simulink model "nav22"  (R2020a)
settings: Solver=VariableStepAuto  StartTime=0.0  StopTime=inf  RelTol=1e-3
values from neighbouring files (symbols this model uses):
  chargingStn = [3, 2]    [startup.m]
  L2RTransform = [cos(L2Rtheta), -sin(L2Rtheta), L2Rx ... (first row only)    [startup.m]
  LIVE_MODE = 1    [startup.m]
  loadingStn = [4, 3]    [startup.m]
  logicalMap = simMapPad < 100    [startup.m]
  unloadingStn = [15, 15]    [startup.m]
  W2LOTransform = W2ORTransform/(L2RTransform)    [startup.m]
  wheelBase = 0.4464    [startup.m]
  wheelRadius = 0.1715/2    (= 0.08575)    [startup.m]
undefined symbols (not defined in the file or in its folder): Angular, Linear
libraries: robotlib x6, robotalgslib x1
settings Model: EnablePacing=on  Creator=john  LastModifiedBy=john

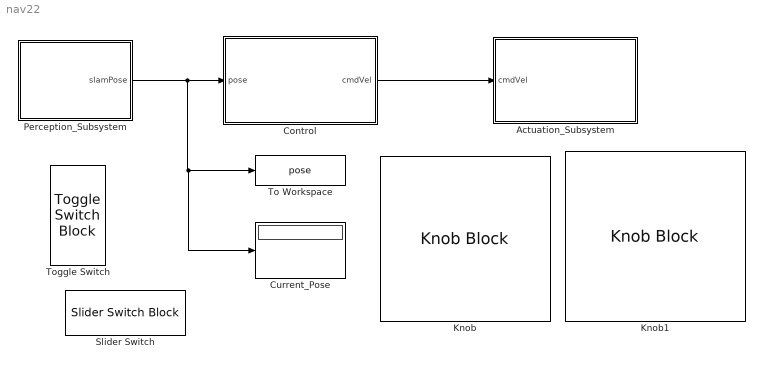
== system nav22 ==
  Actuation_Subsystem : Subsystem
  Control : Subsystem
  Current_Pose : Display
  Knob : KnobBlock  ScaleMin=-5  ScaleMax=5
  Knob1 : KnobBlock  ScaleMin=-1  ScaleMax=1
  Perception_Subsystem : Subsystem
  Slider Switch : SliderSwitchBlock
      settings: Values={{'Off', 'On'}, [0 1]}
  To Workspace : ToWorkspace  VariableName=pose  SaveFormat=Timeseries  SampleTime=-1
  Toggle Switch : ToggleSwitchBlock
      settings: Values={{'Off', 'On'}, [1 0]}
  wires:
  Perception_Subsystem/1(slamPose) -> Current_Pose/1, To Workspace/1, Control/1(pose)
  Control/1(cmdVel) -> Actuation_Subsystem/1(cmdVel)

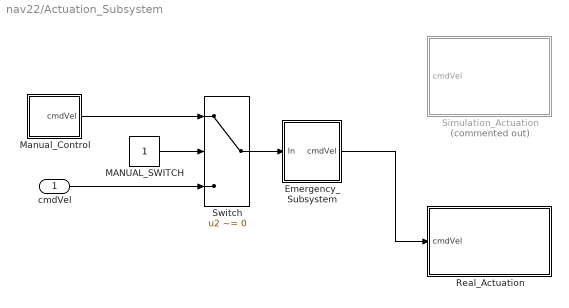
== system nav22/Actuation_Subsystem ==
  cmdVel : Inport
  Emergency_Subsystem : Subsystem
  MANUAL_SWITCH : Constant
  Manual_Control : Subsystem
  Real_Actuation : Subsystem
  Simulation_Actuation : Subsystem  Commented=on
  Switch : Switch  Criteria=u2 ~= 0
  wires:
  cmdVel/1 -> Switch/3
  Manual_Control/1(cmdVel) -> Switch/1
  Switch/1 -> Emergency_Subsystem/1(In)
  Emergency_Subsystem/1(cmdVel) -> Real_Actuation/1(cmdVel)
  MANUAL_SWITCH/1 -> Switch/2

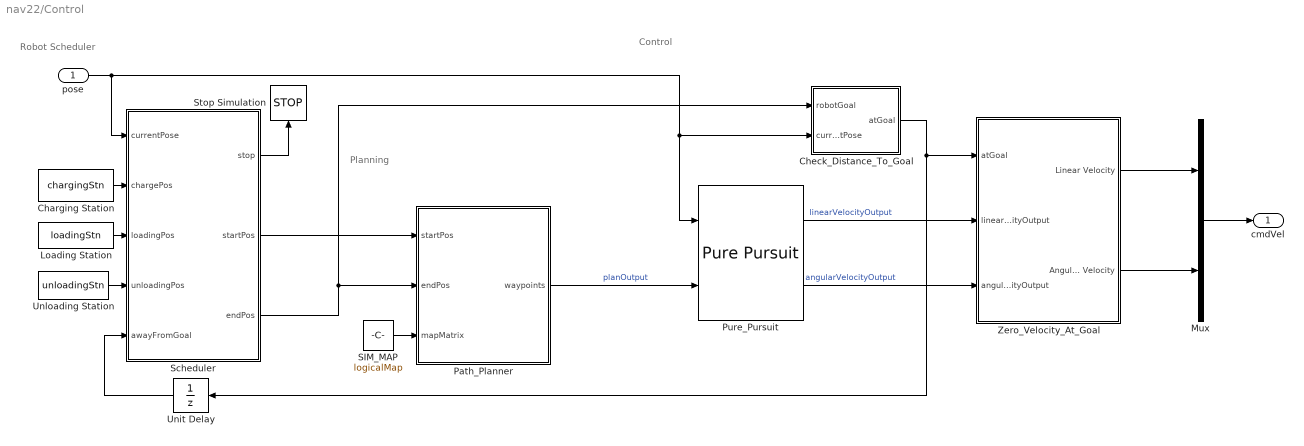
== system nav22/Control ==
  note: Control
  note: Robot Scheduler
  note: Planning
  pose : Inport
  "Charging Station " : Constant  Value=chargingStn  SampleTime=1
  Check_Distance_To_Goal : Subsystem
  Loading Station : Constant  Value=loadingStn
  Mux : Mux  Inputs=2
  Path_Planner : MATLAB Function  TreatAsAtomicUnit=on
  Pure_Pursuit : robotalgslib/Pure Pursuit  DesiredLinearVelocity=1  MaxAngularVelocity=0.5  LookaheadDistance=1  TargetDirPort=off  SimulateUsing=Code generation
  SIM_MAP : Constant  Value=logicalMap  SampleTime=1
  Scheduler : Stateflow chart  TreatAsAtomicUnit=on
  Stop Simulation : Stop
  Unit Delay : UnitDelay  SampleTime=-1  HasFrameUpgradeWarning=on
  Unloading Station : Constant  Value=unloadingStn  SampleTime=1
  Zero_Velocity_At_Goal : Subsystem
  cmdVel : Outport
  wires:
  Check_Distance_To_Goal/1(atGoal) -> Unit Delay/1, Zero_Velocity_At_Goal/1(atGoal)
  "Charging Station "/1 -> Scheduler/2(chargePos)
  Scheduler/2(startPos) -> Path_Planner/1(startPos)
  Unit Delay/1 -> Scheduler/5(awayFromGoal)
  Scheduler/3(endPos) -> Path_Planner/2(endPos), Check_Distance_To_Goal/1(robotGoal)
  Loading Station/1 -> Scheduler/3(loadingPos)
  Pure_Pursuit/2 -> Zero_Velocity_At_Goal/3(angularVelocityOutput)  "angularVelocityOutput"
  pose/1 -> Check_Distance_To_Goal/2(currentPose), Pure_Pursuit/1, Scheduler/1(currentPose)
  Unloading Station/1 -> Scheduler/4(unloadingPos)
  Scheduler/1(stop) -> Stop Simulation/1
  Path_Planner/1(waypoints) -> Pure_Pursuit/2  "planOutput"
  Pure_Pursuit/1 -> Zero_Velocity_At_Goal/2(linearVelocityOutput)  "linearVelocityOutput"
  Zero_Velocity_At_Goal/2(Angular Velocity) -> Mux/2
  Zero_Velocity_At_Goal/1(Linear Velocity) -> Mux/1
  Mux/1 -> cmdVel/1
  SIM_MAP/1 -> Path_Planner/3(mapMatrix)

== system nav22/Perception_Subsystem ==
  SLAM_Subsystem : Subsystem
  slamPose : Outport
  wires:
  SLAM_Subsystem/1(slamPose) -> slamPose/1

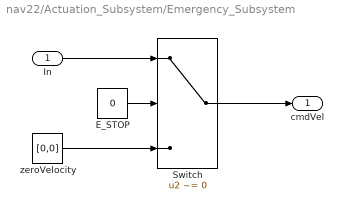
== system nav22/Actuation_Subsystem/Emergency_Subsystem ==
  In : Inport
  E_STOP : Constant  Value=0
  Switch : Switch  Criteria=u2 ~= 0  Threshold=1
  zeroVelocity : Constant  Value=[0,0]
  cmdVel : Outport
  wires:
  Switch/1 -> cmdVel/1
  E_STOP/1 -> Switch/2
  In/1 -> Switch/1
  zeroVelocity/1 -> Switch/3

== system nav22/Actuation_Subsystem/Manual_Control ==
  Mux : Mux  Inputs=2
  angularVel : Constant  Value=-0.007065188519232657
  linearVel : Constant  Value=2.054641124404234
  cmdVel : Outport
  wires:
  linearVel/1 -> Mux/1
  angularVel/1 -> Mux/2
  Mux/1 -> cmdVel/1

== system nav22/Actuation_Subsystem/Real_Actuation ==
  cmdVel : Inport
  Actuator : Subsystem
  Demux : Demux  Outputs=2
  Forward Kinematics : Subsystem
  wires:
  Forward Kinematics/1(leftRpmOut) -> Actuator/1(leftRPM)
  Demux/1 -> Forward Kinematics/1(v_in)
  Forward Kinematics/2(rightRpmOut) -> Actuator/2(rightRPM)
  Demux/2 -> Forward Kinematics/2(w_in)
  cmdVel/1 -> Demux/1

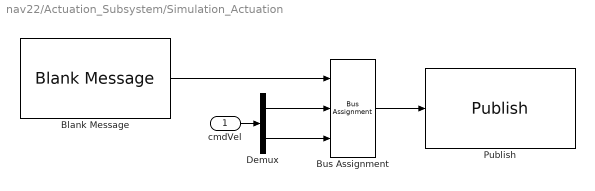
== system nav22/Actuation_Subsystem/Simulation_Actuation ==
  cmdVel : Inport
  Blank Message : robotlib/Blank Message  messageClass=Message  entityType=geometry_msgs/Twist  messageType=geometry_msgs/Twist  SampleTime=inf
  Bus Assignment : BusAssignment  AssignedSignals=Linear.X,Angular.Z
  Demux : Demux  Outputs=2
  Publish : robotlib/Publish  topicSource=Select from ROS network  topic=/cmd_vel  messageType=geometry_msgs/Twist  messageQueueLength=1
  wires:
  Blank Message/1 -> Bus Assignment/1
  Bus Assignment/1 -> Publish/1
  Demux/2 -> Bus Assignment/3
  Demux/1 -> Bus Assignment/2
  cmdVel/1 -> Demux/1

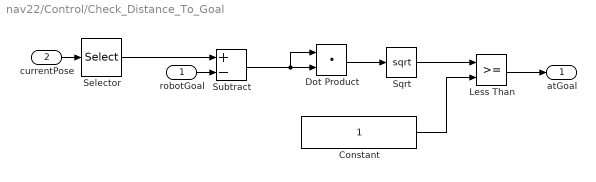
== system nav22/Control/Check_Distance_To_Goal ==
  robotGoal : Inport
  currentPose : Inport  Port=2
  Constant : Constant
  Dot Product : DotProduct  InputSameDT=on  OutDataTypeStr=Inherit: Inherit via internal rule
  Less Than : RelationalOperator  OutDataTypeStr=boolean  RndMeth=Simplest
  Selector : Selector  InputPortWidth=3  IndexOptions=Index vector (dialog)  Indices=[1 2]  OutputSizes=1
  Sqrt : Sqrt  SaturateOnIntegerOverflow=on
  Subtract : Sum  Inputs=+-
  atGoal : Outport
  wires:
  robotGoal/1 -> Subtract/2
  Dot Product/1 -> Sqrt/1
  Constant/1 -> Less Than/2
  currentPose/1 -> Selector/1
  Less Than/1 -> atGoal/1
  Sqrt/1 -> Less Than/1
  Subtract/1 -> Dot Product/1, Dot Product/2
  Selector/1 -> Subtract/1

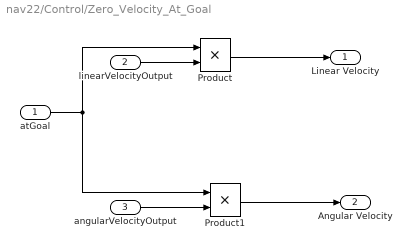
== system nav22/Control/Zero_Velocity_At_Goal ==
  atGoal : Inport
  linearVelocityOutput : Inport  Port=2
  angularVelocityOutput : Inport  Port=3
  Product : Product
  Product1 : Product
  Linear Velocity : Outport  OutDataTypeStr=double
  Angular Velocity : Outport  Port=2  OutDataTypeStr=double
  wires:
  atGoal/1 -> Product1/1, Product/1
  angularVelocityOutput/1 -> Product1/2
  linearVelocityOutput/1 -> Product/2
  Product/1 -> Linear Velocity/1
  Product1/1 -> Angular Velocity/1

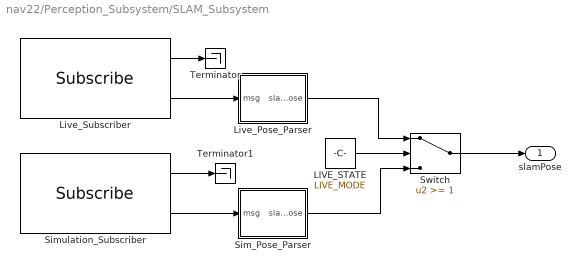
== system nav22/Perception_Subsystem/SLAM_Subsystem ==
  LIVE_STATE : Constant  Value=LIVE_MODE
  Live_Pose_Parser : Subsystem
  Live_Subscriber : robotlib/Subscribe  topicSource=Select from ROS network  topic=/slamware_ros_sdk_server_node/odom  messageType=nav_msgs/Odometry  sampleTime=-1  messageQueueLength=1
  Sim_Pose_Parser : Subsystem
  Simulation_Subscriber : robotlib/Subscribe  topicSource=Select from ROS network  topic=/amcl_pose  messageType=geometry_msgs/PoseWithCovarianceStamped  sampleTime=-1  messageQueueLength=1
  Switch : Switch  Threshold=1
  Terminator : Terminator
  Terminator1 : Terminator
  slamPose : Outport
  wires:
  LIVE_STATE/1 -> Switch/2
  Live_Subscriber/2 -> Live_Pose_Parser/1(msg)
  Simulation_Subscriber/2 -> Sim_Pose_Parser/1(msg)
  Sim_Pose_Parser/1(slamPose) -> Switch/3
  Live_Pose_Parser/1(slamPose) -> Switch/1
  Switch/1 -> slamPose/1
  Simulation_Subscriber/1 -> Terminator1/1
  Live_Subscriber/1 -> Terminator/1

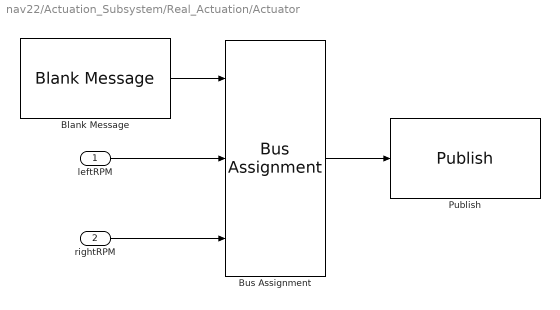
== system nav22/Actuation_Subsystem/Real_Actuation/Actuator ==
  leftRPM : Inport
  rightRPM : Inport  Port=2
  Blank Message : robotlib/Blank Message  messageClass=Message  entityType=geometry_msgs/Twist  messageType=geometry_msgs/Twist  SampleTime=inf
  Bus Assignment : BusAssignment  AssignedSignals=Angular.X,Angular.Y
  Publish : robotlib/Publish  topicSource=Select from ROS network  topic=/zlac8015d/rpm  messageType=geometry_msgs/Twist  messageQueueLength=1
  wires:
  Bus Assignment/1 -> Publish/1
  Blank Message/1 -> Bus Assignment/1
  rightRPM/1 -> Bus Assignment/3
  leftRPM/1 -> Bus Assignment/2

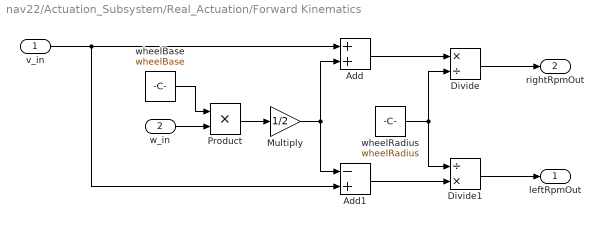
== system nav22/Actuation_Subsystem/Real_Actuation/Forward Kinematics ==
  v_in : Inport
  w_in : Inport  Port=2
  Add : Sum
  Add1 : Sum  Inputs=-+
  Divide : Product  Inputs=*/
  Divide1 : Product  Inputs=/*
  Multiply : Gain  Gain=1/2
  Product : Product
  wheelBase : Constant  Value=wheelBase
  wheelRadius : Constant  Value=wheelRadius
  leftRpmOut : Outport
  rightRpmOut : Outport  Port=2
  wires:
  v_in/1 -> Add1/2, Add/1
  w_in/1 -> Product/2
  wheelBase/1 -> Product/1
  Product/1 -> Multiply/1
  Multiply/1 -> Add/2, Add1/1
  Add1/1 -> Divide1/2
  Add/1 -> Divide/1
  wheelRadius/1 -> Divide1/1, Divide/2
  Divide1/1 -> leftRpmOut/1
  Divide/1 -> rightRpmOut/1

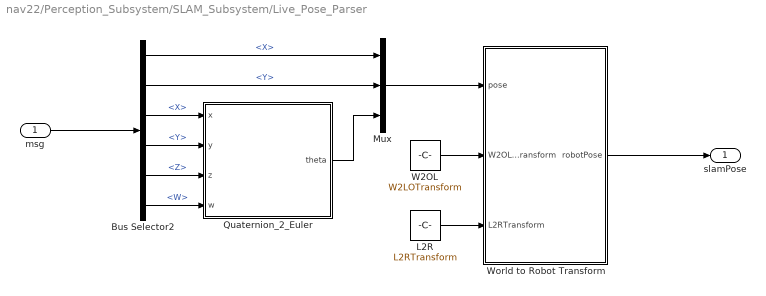
== system nav22/Perception_Subsystem/SLAM_Subsystem/Live_Pose_Parser ==
  msg : Inport
  Bus Selector2 : BusSelector  OutputSignals=Pose.Pose.Position.X,Pose.Pose.Position.Y,Pose.Pose.Orientation.X,Pose.Pose.Orientation.Y,Pose.Pose.Orientation.Z,Pose.Pose.Orientation.W
  L2R : Constant  Value=L2RTransform
  Mux : Mux  Inputs=3
  Quaternion_2_Euler : MATLAB Function  TreatAsAtomicUnit=on
  W2OL : Constant  Value=W2LOTransform
  World to Robot Transform : MATLAB Function  TreatAsAtomicUnit=on
  slamPose : Outport
  wires:
  msg/1 -> Bus Selector2/1
  Bus Selector2/1 -> Mux/1  "<X>"
  Bus Selector2/2 -> Mux/2  "<Y>"
  Bus Selector2/3 -> Quaternion_2_Euler/1(x)  "<X>"
  Bus Selector2/4 -> Quaternion_2_Euler/2(y)  "<Y>"
  Bus Selector2/5 -> Quaternion_2_Euler/3(z)  "<Z>"
  Bus Selector2/6 -> Quaternion_2_Euler/4(w)  "<W>"
  Quaternion_2_Euler/1(theta) -> Mux/3
  Mux/1 -> World to Robot Transform/1(pose)
  World to Robot Transform/1(robotPose) -> slamPose/1
  W2OL/1 -> World to Robot Transform/2(W2OLTransform)
  L2R/1 -> World to Robot Transform/3(L2RTransform)

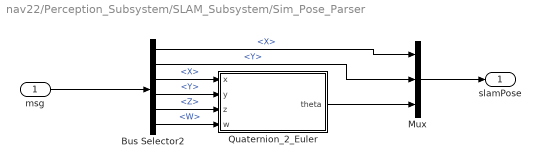
== system nav22/Perception_Subsystem/SLAM_Subsystem/Sim_Pose_Parser ==
  msg : Inport
  Bus Selector2 : BusSelector  OutputSignals=Pose.Pose.Position.X,Pose.Pose.Position.Y,Pose.Pose.Orientation.X,Pose.Pose.Orientation.Y,Pose.Pose.Orientation.Z,Pose.Pose.Orientation.W
  Mux : Mux  Inputs=3
  Quaternion_2_Euler : MATLAB Function  TreatAsAtomicUnit=on
  slamPose : Outport
  wires:
  msg/1 -> Bus Selector2/1
  Mux/1 -> slamPose/1
  Bus Selector2/1 -> Mux/1  "<X>"
  Bus Selector2/2 -> Mux/2  "<Y>"
  Bus Selector2/3 -> Quaternion_2_Euler/1(x)  "<X>"
  Bus Selector2/4 -> Quaternion_2_Euler/2(y)  "<Y>"
  Bus Selector2/5 -> Quaternion_2_Euler/3(z)  "<Z>"
  Bus Selector2/6 -> Quaternion_2_Euler/4(w)  "<W>"
  Quaternion_2_Euler/1(theta) -> Mux/3

== matlab function nav22/Perception_Subsystem/SLAM_Subsystem/Sim_Pose_Parser/Quaternion_2_Euler ==
  data: x input; theta output; y input; z input; w input
function theta = fcn(x, y, z, w)

    euler = quat2eul([x, y, z, w]); 
    
    if sum(isnan(euler)) == 3
        
        euler = ([pi, 0, 0]);
        
    end 
    
theta = euler(1,3);

== matlab function nav22/Control/Path_Planner ==
  settings: updateMethod=DISCRETE
  data: startPos input size=[1 2]; endPos input size=[1 2]; waypoints output size=[500 2]; mapMatrix input
function waypoints = planning(startPos, endPos, mapMatrix)

persistent waypointsInternal
persistent prevStartPos
persistent prevEndPos

% Set constant parameters
maxNumNodes = 500;
robotLength = 0.775;

% Initialize persistent variables that are used downstream
if isempty(prevStartPos)
    prevStartPos = startPos;
end

if isempty(prevEndPos)
    prevEndPos = endPos;
end

isNewPath = (~isequal(prevStartPos, startPos) || ~isequal(prevEndPos, endPos));

if isempty(waypointsInternal) || isNewPath
    % Two conditions in which waypoints must be set: they are not yet
    % initialized, or they are initialized, but the current start and end
    % do not match those used to generate the previous set of waypoints
    [waypointsInternal] = planPath(mapMatrix, maxNumNodes, startPos, endPos);
end

% Update the outputs
waypoints = waypointsInternal;

% Update the persistent variables that indicate previous state
prevStartPos = startPos;
prevEndPos = endPos;

%% Helper Function

function wayPoints = planPath(mapMatrix, maxNodes, startPos, endPos)
    
    % Create a probabilistic roadmap
    map = binaryOccupancyMap(mapMatrix, 1/0.05);
    inflate(map, robotLength/2);
    prm = mobileRobotPRM(map, maxNodes);
    
    % Find a path between two points
    xy = findpath(prm, startPos(:)', endPos(:)');
    wayPoints = repmat(endPos(:)', maxNodes, 1);
    
    % Number of nodes that are actually used
    numNodes = length(xy);
    wayPoints(1:numNodes,:) = xy;    

end

end

== matlab function nav22/Perception_Subsystem/SLAM_Subsystem/Live_Pose_Parser/World to Robot Transform ==
  data: pose input; robotPose output; W2OLTransform input; L2RTransform input
function robotPose = fcn(pose, W2OLTransform, L2RTransform)
    
    % O2L Transform 
    OL2LTransform = [cos(pose(3,1)), -sin(pose(3,1)), pose(1,1);
                    sin(pose(3,1)), cos(pose(3,1)), pose(2,1);
                    0,              0,              1];

    % Calculate World to Robot
    W2RTransform = W2OLTransform*OL2LTransform*L2RTransform; 
    

    % Extract relevant information
robotPose = [W2RTransform(1,3); W2RTransform(2,3); acos(W2RTransform(1,1))];

== matlab function nav22/Perception_Subsystem/SLAM_Subsystem/Live_Pose_Parser/Quaternion_2_Euler ==
  data: x input; theta output; y input; z input; w input
function theta = fcn(x, y, z, w)

    euler = quat2eul([x, y, z, w]); 
    
    if sum(isnan(euler)) == 3
        
        euler = ([pi, 0, 0]);
        
    end 
    
theta = euler(1,3);

== stateflow chart nav22/Control/Scheduler ==
  settings: sampleTime=0.01
  state Unloading
    entry, during:
    endPos = unloadingPos';
  state Loading
    entry,during:
    endPos = loadingPos';
  state Charging
    entry, during:
    endPos = chargePos';
  (default) -> Loading : {startPos = chargePos';}
  Loading -> Unloading : [~awayFromGoal && after(stopDelay, tick)]
      |
      | {startPos = currentPose(1:2)';}
  Unloading -> Charging : [~awayFromGoal  && after(20, tick)]
      | {startPos = currentPose(1:2)';}
  Charging -> (junction 201) : [~awayFromGoal]{stop = 1;}
  data: currentPose input; stop output =0; chargePos input size=[2 1]; loadingPos input size=[2 1]; unloadingPos input size=[2 1]; startPos output size=[1, 2]; endPos output size=[1, 2]; awayFromGoal input; stopDelay local =5
